simulink model "SimulinkschaltbildTeil1"  (R2014b)
settings: Solver=ode45  StartTime=0.0  StopTime=0.2  RelTol=1e-3
settings Model: Creator=Florian  LastModifiedBy=Florian

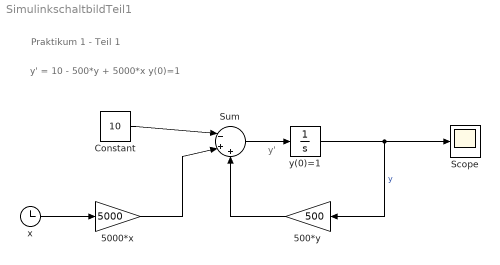
== system SimulinkschaltbildTeil1 ==
  note: Praktikum 1 - Teil 1
  note: y'
  note: y' = 10 - 500*y + 5000*x y(0)=1
  500*y : Gain  Gain=500
  5000*x : Gain  Gain=5000
  Constant : Constant  Value=10
  Scope : Scope
  Sum : Sum  Inputs=|-++
  x : Clock
  y(0)=1 : Integrator
  wires:
  Sum/1 -> y(0)=1/1
  y(0)=1/1 -> Scope/1, 500*y/1  "y"
  Constant/1 -> Sum/1
  5000*x/1 -> Sum/2
  x/1 -> 5000*x/1
  500*y/1 -> Sum/3
